simulink model "tank33v3"  (R2014b)
settings: Solver=ode45  StartTime=0.0  StopTime=100  RelTol=1e-3
model workspace (MAT data in the model file):
  g = 9.81
  r01 = 0.0027
  r11 = 0.053
  r02 = 0.003
  r12 = 0.05
  r21 = 0.055
  H1 = 0.118
settings Model: Creator=jsandoval  LastModifiedBy=jsandoval

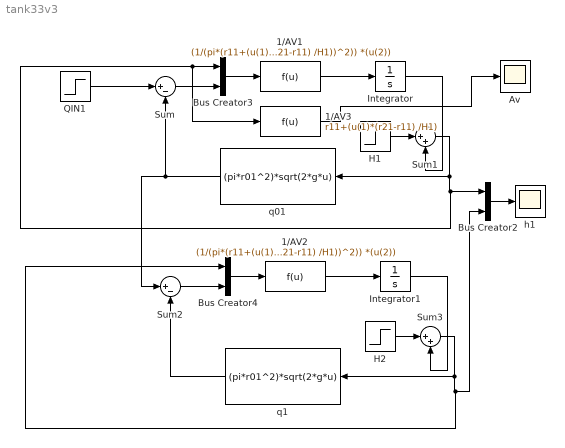
== system tank33v3 ==
  1/AV1 : Fcn  Expr=(1/(pi*(r11+(u(1)*(r21-r11) /H1))^2)) *(u(2))
  1/AV2 : Fcn  Expr=(1/(pi*(r11+(u(1)*(r21-r11) /H1))^2)) *(u(2))
  1/AV3 : Fcn  Expr=r11+(u(1)*(r21-r11) /H1)
  "Av " : Scope
      settings: TimeRange=300  YMin=-0.08  YMax=0.06
  Bus Creator2 : BusCreator  Inputs=2
  Bus Creator3 : BusCreator  Inputs=2
  Bus Creator4 : BusCreator  Inputs=2
  H1 : Step  Time=10  Before=.118  After=.118  SampleTime=1
  H2 : Step  Time=10  Before=.118  After=.118  SampleTime=1
  Integrator : Integrator
  Integrator1 : Integrator
  QIN1 : Step  After=0  SampleTime=1
  Sum : Sum  Inputs=|+-
  Sum1 : Sum  Inputs=|++
  Sum2 : Sum  Inputs=|+-
  Sum3 : Sum  Inputs=|++
  h1 : Scope
      settings: TimeRange=300  YMin=-0.08  YMax=0.06
  q01 : Fcn  Expr=(pi*r01^2)*sqrt(2*g*u)
  q1 : Fcn  Expr=(pi*r01^2)*sqrt(2*g*u)
  wires:
  Sum1/1 -> 1/AV3/1, Bus Creator3/1, Bus Creator2/1, q01/1
  H1/1 -> Sum1/1
  Integrator/1 -> Sum1/2
  q01/1 -> Sum2/1, Sum/2
  Sum/1 -> Bus Creator3/2
  1/AV1/1 -> Integrator/1
  Bus Creator3/1 -> 1/AV1/1
  QIN1/1 -> Sum/1
  Sum3/1 -> Bus Creator2/2, Bus Creator4/1, q1/1
  H2/1 -> Sum3/1
  Integrator1/1 -> Sum3/2
  q1/1 -> Sum2/2
  Sum2/1 -> Bus Creator4/2
  1/AV2/1 -> Integrator1/1
  Bus Creator4/1 -> 1/AV2/1
  Bus Creator2/1 -> h1/1
  1/AV3/1 -> "Av "/1
